simulink model "FTs"  (R2023b)
settings: Solver=VariableStepAuto  StartTime=0.0  StopTime=10.0  RelTol=1e-3
libraries: simulink_extras x1
settings Model: Creator=rafin  LastModifiedBy=rafin

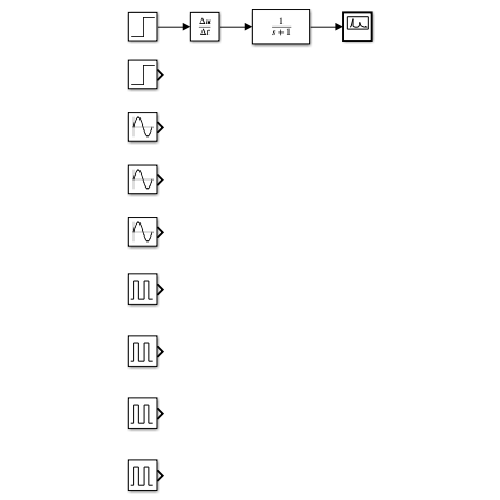
[thumbnail: Simulink's stored preview of the top-level diagram]
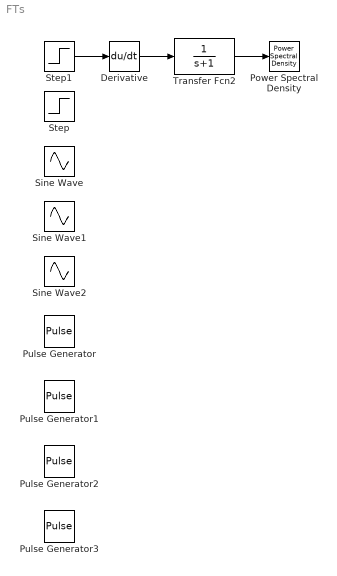
== system FTs ==
  Derivative : Derivative
  Power Spectral Density : simulink_extras/Additional Sinks/Power Spectral Density  npts=128  fftpts=512  HowOften=64  sampleT=0.1
  Pulse Generator : DiscretePulseGenerator  PulseType=Time based  Period=1.5  PulseWidth=10
  Pulse Generator1 : DiscretePulseGenerator  PulseType=Time based  Period=1.5  PulseWidth=80
  Pulse Generator2 : DiscretePulseGenerator  PulseType=Time based  Period=0.4  PulseWidth=10
  Pulse Generator3 : DiscretePulseGenerator  PulseType=Time based  Period=0.4  PulseWidth=80
  Sine Wave : Sin  Frequency=3  SampleTime=0
  Sine Wave1 : Sin  Frequency=10  SampleTime=0
  Sine Wave2 : Sin  Frequency=25  SampleTime=0
  Step : Step  SampleTime=0
  Step1 : Step  SampleTime=0
  Transfer Fcn2 : TransferFcn  Denominator=[1 1]
  wires:
  Step1/1 -> Derivative/1
  Derivative/1 -> Transfer Fcn2/1
  Transfer Fcn2/1 -> Power Spectral Density/1
